simulink model "BFE_TestHarness"  (Simulink 8.6)
settings: Solver=FixedStepDiscrete  StartTime=0.0  StopTime=3  FixedStep=Ts  RelTol=1e-3
PreLoadFcn:
  | addpath('MBD_Tests')
  | 
  | load('Workspace\EnvVar.mat')
  | run('MBD_Tests\MBD_tests_init.m')
  | if exist('tl_preloadfcn','file'), tl_preloadfcn(gcs,402); end
PostLoadFcn:
  | if exist('tl_postloadfcn','file'), tl_postloadfcn(gcs,402); end
InitFcn:
  | if exist('tlds_init','file'), tlds_init(gcs); end
StartFcn:
  | if exist('tlds_start','file'), tlds_start(gcs); end
StopFcn:
  | if exist('tlds_stop','file'), tlds_stop(gcs); end
undefined symbols (not defined in the file): ddv, Ts, u2, u3, u4
libraries: tllib x11, simulink x8, LIB_TF_G_111 x2, LIB_TF_G_12_StepControl x2, LIB_TF_G_112 x1, LIB_TF_G_113 x1
(part 9 of 17)

== system BFE_TestHarness/BFE_AC_BeltFunctionExecution/Subsystem/BFE_AC_BeltFunctionExecution/BFE_AC_BeltFunctionExecution/BFE_runExecuteStandardSteps/ExecuteStandardSteps/SubsystemConvertOrderToMotorPower/Init_Error_Calculation ==
  bIsPRevStepHP : Inport  RequirementInfo={} %GIDa_3aeca3b8_c2ea_4c02_8ac4_92ccbe5190c0
  s8OldPWM : Inport  RequirementInfo={} %GIDa_90f46303_ced5_474c_93d6_f92ab99d1bda  Port=2
  s32OldErrorInteger : Inport  RequirementInfo={} %GIDa_3b3164d8_b308_429e_9a70_7366f48c17f1  Port=3
  Constant : Constant  Value=64  mask(TL_Constant){data={'date',735951.66853295139}}
      settings: CopyFcn=if exist('tl_reset_reviewflag','file')==2,tl_reset_reviewflag(gcbh);end  DeleteFcn=if exist('delete_tlblock','file')==2,delete_tlblock(gcbh);end  NameChangeFcn=if exist('rename_tlblock','file')==2,rename_tlblock(gcbh);end  OpenFcn=if exist('tl_open_blockdlg','file')==2,tl_open_blockdlg(gcbh);else,open_system(gcbh,'parameter');end
      mask Help: eval(['if exist(''tl_online_help'',''file'') == 2, tl_online_help(''Topic'',''TL_Constant''),else, web([''jar:file:///'',matlabroot,''/help/toolbox/simulink/help.jar!/slref/' lower(get_param(gcbh,'Blocktype')) '.html''], ''-helpbrowser''),end'])
      mask Display: plot([-0.05, 1.05, NaN, -0.05, 1.05],[.01, .01, NaN, .99, .99])
  KU16_INIT_INT_ERR_AFTER_HP_STEP : Constant  RequirementInfo={} %GIDa_0c6897e5_41ba_4ffa_a647_dc1e963ab64a  Value=ddv('BFE_Config_Data/KU16_INIT_INT_ERR_AFTER_HP_STEP')  OutDataTypeStr=uint16  mask(TL_Constant){data={'output',{'variable','BFE_Config_Data/KU16_INIT_INT_ERR_AFTER_HP_STEP'},'date',735951.66853256943}}
      settings: CopyFcn=if exist('tl_reset_reviewflag','file')==2,tl_reset_reviewflag(gcbh);end  DeleteFcn=if exist('delete_tlblock','file')==2,delete_tlblock(gcbh);end  NameChangeFcn=if exist('rename_tlblock','file')==2,rename_tlblock(gcbh);end  OpenFcn=if exist('tl_open_blockdlg','file')==2,tl_open_blockdlg(gcbh);else,open_system(gcbh,'parameter');end
      mask Help: eval(['if exist(''tl_online_help'',''file'') == 2, tl_online_help(''Topic'',''TL_Constant''),else, web([''jar:file:///'',matlabroot,''/help/toolbox/simulink/help.jar!/slref/' lower(get_param(gcbh,'Blocktype')) '.html''], ''-helpbrowser''),end'])
      mask Display: plot([-0.05, 1.05, NaN, -0.05, 1.05],[.01, .01, NaN, .99, .99])
  Logical Operator : Logic  RequirementInfo={} %GIDa_e9ae38f0_28a3_485d_bbad_fe83290044bf  Operator=NOT  Inputs=1  AllPortsSameDT=off  OutDataTypeStr=boolean  mask(TL_LogicalOperator){data={'date',735951.66853221064}}
      settings: DeleteFcn=if exist('delete_tlblock','file')==2,delete_tlblock(gcbh);end  NameChangeFcn=if exist('rename_tlblock','file')==2,rename_tlblock(gcbh);end  OpenFcn=if exist('tl_open_blockdlg','file')==2,tl_open_blockdlg(gcbh);else,open_system(gcbh,'parameter');end
      mask Help: eval(['if exist(''tl_online_help'',''file'') == 2, tl_online_help(''Topic'',''TL_LogicalOperator''),else, web([''jar:file:///'',matlabroot,''/help/toolbox/simulink/help.jar!/slref/' lower(get_param(gcbh,'Blocktype')) '.html''], ''-helpbrowser''),end'])
      mask Display: plot([-0.05, 1.05, NaN, -0.05, 1.05],[.01, .01, NaN, .99, .99])
  Product : Product  RequirementInfo={} %GIDa_8a9d49ec_e92b_4899_920d_3eb12938c5eb  Inputs=**  RndMeth=Zero  mask(TL_Product){data={'output',{'type','Int32'},'date',735951.66853192134}}
      settings: CopyFcn=if exist('tl_reset_reviewflag','file')==2,tl_reset_reviewflag(gcbh);end  DeleteFcn=if exist('delete_tlblock','file')==2,delete_tlblock(gcbh);end  NameChangeFcn=if exist('rename_tlblock','file')==2,rename_tlblock(gcbh);end  OpenFcn=if exist('tl_open_blockdlg','file')==2,tl_open_blockdlg(gcbh);else,open_system(gcbh,'parameter');end
      mask Help: eval(['if exist(''tl_online_help'',''file'') == 2, tl_online_help(''Topic'',''TL_Product''),else, web([''jar:file:///'',matlabroot,''/help/toolbox/simulink/help.jar!/slref/' lower(get_param(gcbh,'Blocktype')) '.html''], ''-helpbrowser''),end'])
      mask Display: plot([-0.05, 1.05, NaN, -0.05, 1.05],[.01, .01, NaN, .99, .99])
  Product1 : Product  Inputs=*/  RndMeth=Zero  mask(TL_Product){data={'date',735951.66853155091}}
      settings: CopyFcn=if exist('tl_reset_reviewflag','file')==2,tl_reset_reviewflag(gcbh);end  DeleteFcn=if exist('delete_tlblock','file')==2,delete_tlblock(gcbh);end  NameChangeFcn=if exist('rename_tlblock','file')==2,rename_tlblock(gcbh);end  OpenFcn=if exist('tl_open_blockdlg','file')==2,tl_open_blockdlg(gcbh);else,open_system(gcbh,'parameter');end
      mask Help: eval(['if exist(''tl_online_help'',''file'') == 2, tl_online_help(''Topic'',''TL_Product''),else, web([''jar:file:///'',matlabroot,''/help/toolbox/simulink/help.jar!/slref/' lower(get_param(gcbh,'Blocktype')) '.html''], ''-helpbrowser''),end'])
      mask Display: plot([-0.05, 1.05, NaN, -0.05, 1.05],[.01, .01, NaN, .99, .99])
  Switch2 : Switch  RequirementInfo={} %GIDa_7eaf5a01_1953_49b8_89c4_2db1d6eb7e42  Criteria=u2 ~= 0  mask(TL_Switch){data={'output',{'type','Int32'},'date',735951.66853114578}}
      settings: CopyFcn=if exist('tl_reset_reviewflag','file')==2,tl_reset_reviewflag(gcbh);end  DeleteFcn=if exist('delete_tlblock','file')==2,delete_tlblock(gcbh);end  NameChangeFcn=if exist('rename_tlblock','file')==2,rename_tlblock(gcbh);end  OpenFcn=if exist('tl_open_blockdlg','file')==2,tl_open_blockdlg(gcbh);else,open_system(gcbh,'parameter');end
      mask Help: eval(['if exist(''tl_online_help'',''file'') == 2, tl_online_help(''Topic'',''TL_Switch''),else, web([''jar:file:///'',matlabroot,''/help/toolbox/simulink/help.jar!/slref/' lower(get_param(gcbh,'Blocktype')) '.html''], ''-helpbrowser''),end'])
      mask Display: plot([-0.05, 1.05, NaN, -0.05, 1.05],[.01, .01, NaN, .99, .99])
  s32OldErrorIntegerOut : Outport  RequirementInfo={} %GIDa_0e251ad7_27d7_4147_9d0f_3aab0ebc726c
  wires:
  s32OldErrorInteger/1 -> Switch2/1
  bIsPRevStepHP/1 -> Logical Operator/1
  Logical Operator/1 -> Switch2/2
  Switch2/1 -> s32OldErrorIntegerOut/1
  Product/1 -> Switch2/3
  KU16_INIT_INT_ERR_AFTER_HP_STEP/1 -> Product/2
  Product1/1 -> Product/1
  s8OldPWM/1 -> Product1/1
  Constant/1 -> Product1/2

== system BFE_TestHarness/BFE_AC_BeltFunctionExecution/Subsystem/BFE_AC_BeltFunctionExecution/BFE_AC_BeltFunctionExecution/BFE_runExecuteStandardSteps/ExecuteStandardSteps/SubsystemConvertOrderToMotorPower/ManageIntegerErrorReset ==
  u8OrderType : Inport  RequirementInfo={} %GIDa_8549e3bb_6e62_49c5_b285_24fb3bfbc57d
  s32IntegerErrorBeforeFiltering : Inport  RequirementInfo={} %GIDa_94248635_d0d9_4096_9756_d2821aac4d1d  Port=2
  Constant : Constant  RequirementInfo={} %GIDa_400b47d7_22f6_4b23_999f_d1b51fb3a630  Value=ddv('BFE/Step_Def/KU8_NO_STEP_TYPE')  OutDataTypeStr=uint8  mask(TL_Constant){data={'output',{'variable','BFE/Step_Def/KU8_NO_STEP_TYPE'},'date',735951.66853064811}}
      settings: AttributesFormatString=KUC_ORDER_NO_STEP  CopyFcn=if exist('tl_reset_reviewflag','file')==2,tl_reset_reviewflag(gcbh);end  DeleteFcn=if exist('delete_tlblock','file')==2,delete_tlblock(gcbh);end  NameChangeFcn=if exist('rename_tlblock','file')==2,rename_tlblock(gcbh);end  OpenFcn=if exist('tl_open_blockdlg','file')==2,tl_open_blockdlg(gcbh);else,open_system(gcbh,'parameter');end
      mask Help: eval(['if exist(''tl_online_help'',''file'') == 2, tl_online_help(''Topic'',''TL_Constant''),else, web([''jar:file:///'',matlabroot,''/help/toolbox/simulink/help.jar!/slref/' lower(get_param(gcbh,'Blocktype')) '.html''], ''-helpbrowser''),end'])
      mask Display: plot([-0.05, 1.05, NaN, -0.05, 1.05],[.01, .01, NaN, .99, .99])
  Constant1 : Constant  RequirementInfo={} %GIDa_60b49a3c_45d1_477a_9f0e_42be2507b875  Value=ddv('Common/KU16_ZERO')  OutDataTypeStr=uint16  mask(TL_Constant){data={'output',{'variable','Common/KU16_ZERO'},'date',735951.66853027779}}
      settings: AttributesFormatString=0  CopyFcn=if exist('tl_reset_reviewflag','file')==2,tl_reset_reviewflag(gcbh);end  DeleteFcn=if exist('delete_tlblock','file')==2,delete_tlblock(gcbh);end  NameChangeFcn=if exist('rename_tlblock','file')==2,rename_tlblock(gcbh);end  OpenFcn=if exist('tl_open_blockdlg','file')==2,tl_open_blockdlg(gcbh);else,open_system(gcbh,'parameter');end
      mask Help: eval(['if exist(''tl_online_help'',''file'') == 2, tl_online_help(''Topic'',''TL_Constant''),else, web([''jar:file:///'',matlabroot,''/help/toolbox/simulink/help.jar!/slref/' lower(get_param(gcbh,'Blocktype')) '.html''], ''-helpbrowser''),end'])
      mask Display: plot([-0.05, 1.05, NaN, -0.05, 1.05],[.01, .01, NaN, .99, .99])
  Constant2 : Constant  RequirementInfo={} %GIDa_d35160b3_7e05_486a_a35e_53ff5ad5257b  Value=ddv('Sampling_Freq/KUS_MOTOR_PERIOD')  OutDataTypeStr=uint16  mask(TL_Constant){data={'output',{'variable','Sampling_Freq/KUS_MOTOR_PERIOD'},'date',735951.66852989583}}
      settings: AttributesFormatString=KUS_MOTOR_PERIOD  CopyFcn=if exist('tl_reset_reviewflag','file')==2,tl_reset_reviewflag(gcbh);end  DeleteFcn=if exist('delete_tlblock','file')==2,delete_tlblock(gcbh);end  NameChangeFcn=if exist('rename_tlblock','file')==2,rename_tlblock(gcbh);end  OpenFcn=if exist('tl_open_blockdlg','file')==2,tl_open_blockdlg(gcbh);else,open_system(gcbh,'parameter');end
      mask Help: eval(['if exist(''tl_online_help'',''file'') == 2, tl_online_help(''Topic'',''TL_Constant''),else, web([''jar:file:///'',matlabroot,''/help/toolbox/simulink/help.jar!/slref/' lower(get_param(gcbh,'Blocktype')) '.html''], ''-helpbrowser''),end'])
      mask Display: plot([-0.05, 1.05, NaN, -0.05, 1.05],[.01, .01, NaN, .99, .99])
  Constant3 : Constant  RequirementInfo={} %GIDa_93e02d8c_4049_4a05_a6b4_77b5e0e5f5bc  Value=ddv('BFE_Config_Data/KUS_LATENCY_TIME')  OutDataTypeStr=uint16  mask(TL_Constant){data={'output',{'variable','BFE_Config_Data/KUS_LATENCY_TIME'},'date',735951.66852952552}}
      settings: AttributesFormatString=KUS_LATENCY_TIME  CopyFcn=if exist('tl_reset_reviewflag','file')==2,tl_reset_reviewflag(gcbh);end  DeleteFcn=if exist('delete_tlblock','file')==2,delete_tlblock(gcbh);end  NameChangeFcn=if exist('rename_tlblock','file')==2,rename_tlblock(gcbh);end  OpenFcn=if exist('tl_open_blockdlg','file')==2,tl_open_blockdlg(gcbh);else,open_system(gcbh,'parameter');end
      mask Help: eval(['if exist(''tl_online_help'',''file'') == 2, tl_online_help(''Topic'',''TL_Constant''),else, web([''jar:file:///'',matlabroot,''/help/toolbox/simulink/help.jar!/slref/' lower(get_param(gcbh,'Blocktype')) '.html''], ''-helpbrowser''),end'])
      mask Display: plot([-0.05, 1.05, NaN, -0.05, 1.05],[.01, .01, NaN, .99, .99])
  Constant4 : Constant  RequirementInfo={} %GIDa_677fe65a_1a86_4eeb_a304_f896904fa8d3  Value=ddv('Common/KS32_ZERO')  OutDataTypeStr=int32  mask(TL_Constant){data={'output',{'variable','Common/KS32_ZERO'},'date',735951.66852913192}}
      settings: AttributesFormatString=0  CopyFcn=if exist('tl_reset_reviewflag','file')==2,tl_reset_reviewflag(gcbh);end  DeleteFcn=if exist('delete_tlblock','file')==2,delete_tlblock(gcbh);end  NameChangeFcn=if exist('rename_tlblock','file')==2,rename_tlblock(gcbh);end  OpenFcn=if exist('tl_open_blockdlg','file')==2,tl_open_blockdlg(gcbh);else,open_system(gcbh,'parameter');end
      mask Help: eval(['if exist(''tl_online_help'',''file'') == 2, tl_online_help(''Topic'',''TL_Constant''),else, web([''jar:file:///'',matlabroot,''/help/toolbox/simulink/help.jar!/slref/' lower(get_param(gcbh,'Blocktype')) '.html''], ''-helpbrowser''),end'])
      mask Display: plot([-0.05, 1.05, NaN, -0.05, 1.05],[.01, .01, NaN, .99, .99])
  Relational Operator : RelationalOperator  RequirementInfo={} %GIDa_8dc24057_5624_4d83_81c1_9cda726f5202  Operator===  OutDataTypeStr=boolean  mask(TL_RelationalOperator){data={'date',735951.6685287616}}
      settings: DeleteFcn=if exist('delete_tlblock','file')==2,delete_tlblock(gcbh);end  NameChangeFcn=if exist('rename_tlblock','file')==2,rename_tlblock(gcbh);end  OpenFcn=if exist('tl_open_blockdlg','file')==2,tl_open_blockdlg(gcbh);else,open_system(gcbh,'parameter');end
      mask Help: eval(['if exist(''tl_online_help'',''file'') == 2, tl_online_help(''Topic'',''TL_RelationalOperator''),else, web([''jar:file:///'',matlabroot,''/help/toolbox/simulink/help.jar!/slref/' lower(get_param(gcbh,'Blocktype')) '.html''], ''-helpbrowser''),end'])
      mask Display: plot([-0.05, 1.05, NaN, -0.05, 1.05],[.01, .01, NaN, .99, .99])
  Relational Operator1 : RelationalOperator  RequirementInfo={} %GIDa_358a1e32_d0c5_4061_86ff_eee2b1d5aee8  Operator===  OutDataTypeStr=boolean  mask(TL_RelationalOperator){data={'date',735951.668528507}}
      settings: DeleteFcn=if exist('delete_tlblock','file')==2,delete_tlblock(gcbh);end  NameChangeFcn=if exist('rename_tlblock','file')==2,rename_tlblock(gcbh);end  OpenFcn=if exist('tl_open_blockdlg','file')==2,tl_open_blockdlg(gcbh);else,open_system(gcbh,'parameter');end
      mask Help: eval(['if exist(''tl_online_help'',''file'') == 2, tl_online_help(''Topic'',''TL_RelationalOperator''),else, web([''jar:file:///'',matlabroot,''/help/toolbox/simulink/help.jar!/slref/' lower(get_param(gcbh,'Blocktype')) '.html''], ''-helpbrowser''),end'])
      mask Display: plot([-0.05, 1.05, NaN, -0.05, 1.05],[.01, .01, NaN, .99, .99])
  Saturation : Saturate  RequirementInfo={} %GIDa_0b354fed_29ce_4153_9483_4349c0983084  UpperLimit=ddv('BFE_Config_Data/KUS_LATENCY_TIME')  LowerLimit=ddv('Common/KU16_ZERO')  mask(TL_Saturate){data={'output',{'type','UInt16'},'lowerlimit',{'variable','Common/KU16_ZERO'},'upperlimit',{'variable','BFE_Config_Data/KUS_LATENCY_TIME'},'date',735951.66852819442}}
      settings: CopyFcn=if exist('tl_reset_reviewflag','file')==2,tl_reset_reviewflag(gcbh);end  DeleteFcn=if exist('delete_tlblock','file')==2,delete_tlblock(gcbh);end  NameChangeFcn=if exist('rename_tlblock','file')==2,rename_tlblock(gcbh);end  OpenFcn=if exist('tl_open_blockdlg','file')==2,tl_open_blockdlg(gcbh);else,open_system(gcbh,'parameter');end
      settings: AttributesFormatString=|
      | Lower limit = %<LowerLimit>
      | Upper limit = %<UpperLimit>
      mask Help: eval(['if exist(''tl_online_help'',''file'') == 2, tl_online_help(''Topic'',''TL_Saturate''),else, web([''jar:file:///'',matlabroot,''/help/toolbox/simulink/help.jar!/slref/' lower(get_param(gcbh,'Blocktype')) '.html''], ''-helpbrowser''),end'])
      mask Display: plot([-0.05, 1.05, NaN, -0.05, 1.05],[.01, .01, NaN, .99, .99])
  Sum : Sum  RequirementInfo={} %GIDa_3d53df66_2771_419d_a11b_8bf48d1e7499  mask(TL_Sum){data={'output',{'type','UInt16'},'date',735951.66852752317}}
      settings: CopyFcn=if exist('tl_reset_reviewflag','file')==2,tl_reset_reviewflag(gcbh);end  DeleteFcn=if exist('delete_tlblock','file')==2,delete_tlblock(gcbh);end  NameChangeFcn=if exist('rename_tlblock','file')==2,rename_tlblock(gcbh);end  OpenFcn=if exist('tl_open_blockdlg','file')==2,tl_open_blockdlg(gcbh);else,open_system(gcbh,'parameter');end
      mask Help: eval(['if exist(''tl_online_help'',''file'') == 2, tl_online_help(''Topic'',''TL_Sum''),else, web([''jar:file:///'',matlabroot,''/help/toolbox/simulink/help.jar!/slref/' lower(get_param(gcbh,'Blocktype')) '.html''], ''-helpbrowser''),end'])
      mask Display: plot([-0.05, 1.05, NaN, -0.05, 1.05],[.01, .01, NaN, .99, .99])
  Switch : Switch  RequirementInfo={} %GIDa_fc0b4065_c48a_495e_8057_422aaf68c743  Criteria=u2 ~= 0  mask(TL_Switch){data={'output',{'type','UInt16'},'date',735951.66852712957}}
      settings: CopyFcn=if exist('tl_reset_reviewflag','file')==2,tl_reset_reviewflag(gcbh);end  DeleteFcn=if exist('delete_tlblock','file')==2,delete_tlblock(gcbh);end  NameChangeFcn=if exist('rename_tlblock','file')==2,rename_tlblock(gcbh);end  OpenFcn=if exist('tl_open_blockdlg','file')==2,tl_open_blockdlg(gcbh);else,open_system(gcbh,'parameter');end
      mask Help: eval(['if exist(''tl_online_help'',''file'') == 2, tl_online_help(''Topic'',''TL_Switch''),else, web([''jar:file:///'',matlabroot,''/help/toolbox/simulink/help.jar!/slref/' lower(get_param(gcbh,'Blocktype')) '.html''], ''-helpbrowser''),end'])
      mask Display: plot([-0.05, 1.05, NaN, -0.05, 1.05],[.01, .01, NaN, .99, .99])
  Switch1 : Switch  RequirementInfo={} %GIDa_8f433719_feec_41c9_b899_87ec8cd62b2c  Criteria=u2 ~= 0  mask(TL_Switch){data={'output',{'type','Int32'},'date',735951.6685265972}}
      settings: CopyFcn=if exist('tl_reset_reviewflag','file')==2,tl_reset_reviewflag(gcbh);end  DeleteFcn=if exist('delete_tlblock','file')==2,delete_tlblock(gcbh);end  NameChangeFcn=if exist('rename_tlblock','file')==2,rename_tlblock(gcbh);end  OpenFcn=if exist('tl_open_blockdlg','file')==2,tl_open_blockdlg(gcbh);else,open_system(gcbh,'parameter');end
      mask Help: eval(['if exist(''tl_online_help'',''file'') == 2, tl_online_help(''Topic'',''TL_Switch''),else, web([''jar:file:///'',matlabroot,''/help/toolbox/simulink/help.jar!/slref/' lower(get_param(gcbh,'Blocktype')) '.html''], ''-helpbrowser''),end'])
      mask Display: plot([-0.05, 1.05, NaN, -0.05, 1.05],[.01, .01, NaN, .99, .99])
  Unit Delay : UnitDelay  RequirementInfo={} %GIDa_8c292399_951b_41af_8b19_51277957374b  SampleTime=-1  mask(TL_UnitDelay){data={'output',{'type','UInt16'},'state',{'name','X_u16CntErrorReset','type','UInt16'},'date',735951.66852607636}}
      settings: CopyFcn=if exist('tl_reset_reviewflag','file')==2,tl_reset_reviewflag(gcbh);end  DeleteFcn=if exist('delete_tlblock','file')==2,delete_tlblock(gcbh);end  NameChangeFcn=if exist('rename_tlblock','file')==2,rename_tlblock(gcbh);end  OpenFcn=if exist('tl_open_blockdlg','file')==2,tl_open_blockdlg(gcbh);else,open_system(gcbh,'parameter');end
      mask Help: eval(['if exist(''tl_online_help'',''file'') == 2, tl_online_help(''Topic'',''TL_UnitDelay''),else, web([''jar:file:///'',matlabroot,''/help/toolbox/simulink/help.jar!/slref/' lower(get_param(gcbh,'Blocktype')) '.html''], ''-helpbrowser''),end'])
      mask Display: plot([-0.05, 1.05, NaN, -0.05, 1.05],[.01, .01, NaN, .99, .99])
  s32OldErrorFiltered : Outport  RequirementInfo={} %GIDa_4f4b4710_9940_4364_9238_933101741456
  b8IsNewCycle : Outport  RequirementInfo={} %GIDa_f359d049_9be5_425a_8c81_91d895b874f4  Port=2
  wires:
  u8OrderType/1 -> Relational Operator/1
  Constant/1 -> Relational Operator/2
  Relational Operator/1 -> Switch/2
  Constant1/1 -> Switch/3
  Unit Delay/1 -> Switch/1
  Constant2/1 -> Sum/2
  Switch/1 -> Sum/1
  Sum/1 -> Saturation/1
  Saturation/1 -> Unit Delay/1, Relational Operator1/1
  Constant3/1 -> Relational Operator1/2
  Relational Operator1/1 -> b8IsNewCycle/1, Switch1/2
  s32IntegerErrorBeforeFiltering/1 -> Switch1/3
  Constant4/1 -> Switch1/1
  Switch1/1 -> s32OldErrorFiltered/1

== system BFE_TestHarness/BFE_AC_BeltFunctionExecution/Subsystem/BFE_AC_BeltFunctionExecution/BFE_AC_BeltFunctionExecution/BFE_runExecuteStandardSteps/ExecuteStandardSteps/SubsystemConvertOrderToMotorPower/MotorVoltage_Regulation ==
  lOrderToApply : Inport  RequirementInfo={} %GIDa_276e94c1_4a1d_4441_aa6e_71c39ac6771d
  usBatteryVoltage : Inport  RequirementInfo={} %GIDa_bdb98f1d_8da6_4ac7_8ba3_6dd808cf08bb  Port=2
  Action Port : ActionPort  RequirementInfo={} %GIDa_490740ec_3218_4b5f_9934_5823e2c144e8  ActionType=case
  Battery voltage rescaling : Subsystem  TreatAsAtomicUnit=on
  Consign < Battery voltage => Compute PWM : Subsystem  TreatAsAtomicUnit=on
  Consign > Battery voltage => Saturate to MAX PWM : Subsystem  TreatAsAtomicUnit=on
  If : If  IfExpression=u1
  Implausible order : RelationalOperator  Operator=>  OutDataTypeStr=boolean  mask(TL_RelationalOperator){data={'date',737167.45056728006}}
      settings: DeleteFcn=if exist('delete_tlblock','file')==2,delete_tlblock(gcbh);end  NameChangeFcn=if exist('rename_tlblock','file')==2,rename_tlblock(gcbh);end  OpenFcn=if exist('tl_open_blockdlg','file')==2,tl_open_blockdlg(gcbh);else,open_system(gcbh,'parameter');end
      mask Help: eval(['if exist(''tl_online_help'',''file'') == 2, tl_online_help(''Topic'',''TL_RelationalOperator''),else, web([''jar:file:///'',matlabroot,''/help/toolbox/simulink/help.jar!/slref/' lower(get_param(gcbh,'Blocktype')) '.html''], ''-helpbrowser''),end'])
      mask Display: plot([-0.1, 1.05, NaN, -0.1, 1.05],[.01, .01, NaN, .99, .99]);
  Merge : Merge  mask(TL_Merge){data={'date',737167.47328359948}}
      settings: CopyFcn=if exist('tl_reset_reviewflag') == 2, tl_reset_reviewflag(gcbh); end  DeleteFcn=if exist('delete_tlblock','file')==2,delete_tlblock(gcbh);end  NameChangeFcn=if exist('rename_tlblock','file')==2,rename_tlblock(gcbh);end  OpenFcn=if exist('tl_open_blockdlg','file')==2,tl_open_blockdlg(gcbh);else,open_system(gcbh,'parameter');end
      mask Help: eval(['if exist(''tl_online_help'',''file'') == 2, tl_online_help(''Topic'',''TL_Merge''),else, web([''jar:file:///'',matlabroot,''/help/toolbox/simulink/help.jar!/slref/' lower(get_param(gcbh,'Blocktype')) '.html''], ''-helpbrowser''),end'])
      mask Display: plot([-0.1, 1.05, NaN, -0.1, 1.05],[.01, .01, NaN, .99, .99]);
  RescalerMotorOrder : DataTypeConversion  RequirementInfo={} %GIDa_7ffb3157_f329_4896_ac59_557cf7694e9e  OutDataTypeStr=int16  RndMeth=Zero  mask(TL_Rescaler){data={'output',{'checkmin',1,'checkmax',1},'date',735951.66852125002}}
      settings: DeleteFcn=if exist('delete_tlblock','file')==2,delete_tlblock(gcbh);end  NameChangeFcn=if exist('rename_tlblock','file')==2,rename_tlblock(gcbh);end  OpenFcn=if exist('tl_open_blockdlg','file')==2,tl_open_blockdlg(gcbh);else,open_system(gcbh,'parameter');end
      mask Help: eval(['if exist(''tl_online_help'',''file'') == 2, tl_online_help(''Topic'',''TL_Rescaler''),else, web([''jar:file:///'',matlabroot,''/help/toolbox/simulink/help.jar!/slref/' lower(get_param(gcbh,'Blocktype')) '.html''], ''-helpbrowser''),end'])
      mask Display: plot([-0.05, 1.05, NaN, -0.05, 1.05],[.01, .01, NaN, .99, .99])
  sUnsaturatedMotorPowerOrder : Outport  RequirementInfo={} %GIDa_8479673a_6f27_43fd_8c97_1bdf8f1b517f
  wires:
  RescalerMotorOrder/1 -> sUnsaturatedMotorPowerOrder/1
  lOrderToApply/1 -> Consign > Battery voltage => Saturate to MAX PWM/1(lOrderToApply), Consign < Battery voltage => Compute PWM/1(lOrderToApply), Implausible order/1
  Merge/1 -> RescalerMotorOrder/1
  usBatteryVoltage/1 -> Consign < Battery voltage => Compute PWM/2(usBatteryVoltage), Battery voltage rescaling/1(usBatteryVoltage)
  Battery voltage rescaling/1(usBatteryVoltageScaled) -> Implausible order/2
  Implausible order/1 -> If/1
  If/2 -> Consign < Battery voltage => Compute PWM/Action
  If/1 -> Consign > Battery voltage => Saturate to MAX PWM/Action
  Consign > Battery voltage => Saturate to MAX PWM/1(sUnsaturatedMotorPowerOrder) -> Merge/1
  Consign < Battery voltage => Compute PWM/1(sUnsaturatedMotorPowerOrder) -> Merge/2

== system BFE_TestHarness/BFE_AC_BeltFunctionExecution/Subsystem/BFE_AC_BeltFunctionExecution/BFE_AC_BeltFunctionExecution/BFE_runExecuteStandardSteps/ExecuteStandardSteps/SubsystemConvertOrderToMotorPower/No_Regulation ==
  Action Port : ActionPort  RequirementInfo={} %GIDa_9c14f1c9_1d70_4ac6_acdc_0eeba1f4106a  ActionType=default
  Constant : Constant  RequirementInfo={} %GIDa_3fa52539_92f4_4b6b_8938_fabe1668a03f  Value=ddv('Common/KS16_ZERO')  OutDataTypeStr=int16  mask(TL_Constant){data={'output',{'variable','Common/KS16_ZERO'},'date',735951.66851976851}}
      settings: CopyFcn=if exist('tl_reset_reviewflag','file')==2,tl_reset_reviewflag(gcbh);end  DeleteFcn=if exist('delete_tlblock','file')==2,delete_tlblock(gcbh);end  NameChangeFcn=if exist('rename_tlblock','file')==2,rename_tlblock(gcbh);end  OpenFcn=if exist('tl_open_blockdlg','file')==2,tl_open_blockdlg(gcbh);else,open_system(gcbh,'parameter');end
      mask Help: eval(['if exist(''tl_online_help'',''file'') == 2, tl_online_help(''Topic'',''TL_Constant''),else, web([''jar:file:///'',matlabroot,''/help/toolbox/simulink/help.jar!/slref/' lower(get_param(gcbh,'Blocktype')) '.html''], ''-helpbrowser''),end'])
      mask Display: plot([-0.05, 1.05, NaN, -0.05, 1.05],[.01, .01, NaN, .99, .99])
  Rescaler : DataTypeConversion  RequirementInfo={} %GIDa_7c165c89_8161_486a_8381_b07b38254a18  OutDataTypeStr=int16  SaturateOnIntegerOverflow=on  RndMeth=Zero  mask(TL_Rescaler){data={'date',735951.66851938656}}
      settings: DeleteFcn=if exist('delete_tlblock','file')==2,delete_tlblock(gcbh);end  NameChangeFcn=if exist('rename_tlblock','file')==2,rename_tlblock(gcbh);end  OpenFcn=if exist('tl_open_blockdlg','file')==2,tl_open_blockdlg(gcbh);else,open_system(gcbh,'parameter');end
      mask Help: eval(['if exist(''tl_online_help'',''file'') == 2, tl_online_help(''Topic'',''TL_Rescaler''),else, web([''jar:file:///'',matlabroot,''/help/toolbox/simulink/help.jar!/slref/' lower(get_param(gcbh,'Blocktype')) '.html''], ''-helpbrowser''),end'])
      mask Display: plot([-0.05, 1.05, NaN, -0.05, 1.05],[.01, .01, NaN, .99, .99])
  s16Consign : Outport  RequirementInfo={} %GIDa_00325fa2_2d83_40ec_a061_c69647143619  InitialOutput=0
  wires:
  Constant/1 -> Rescaler/1
  Rescaler/1 -> s16Consign/1

== system BFE_TestHarness/BFE_AC_BeltFunctionExecution/Subsystem/BFE_AC_BeltFunctionExecution/BFE_AC_BeltFunctionExecution/BFE_runExecuteStandardSteps/ExecuteStandardSteps/SubsystemConvertOrderToMotorPower/PWM_Regulation ==
  s32OrderToApply : Inport  RequirementInfo={} %GIDa_80e886a0_f1c3_49a4_98c6_efd74da0210c
  Action Port : ActionPort  RequirementInfo={} %GIDa_d2103cf1_dcab_4113_8a19_04aa9c62073a  ActionType=case
  Arrondi 1/2 lsb : Constant  Value=ddv('BFE/ExecuteStdSteps_Rescaling/KU16_PWM_RSC_NUM')  mask(TL_Constant){data={'output',{'variable','BFE/ExecuteStdSteps_Rescaling/KU16_PWM_RSC_NUM'},'date',735951.6685190741}}
      settings: CopyFcn=if exist('tl_reset_reviewflag','file')==2,tl_reset_reviewflag(gcbh);end  DeleteFcn=if exist('delete_tlblock','file')==2,delete_tlblock(gcbh);end  NameChangeFcn=if exist('rename_tlblock','file')==2,rename_tlblock(gcbh);end  OpenFcn=if exist('tl_open_blockdlg','file')==2,tl_open_blockdlg(gcbh);else,open_system(gcbh,'parameter');end
      mask Help: eval(['if exist(''tl_online_help'',''file'') == 2, tl_online_help(''Topic'',''TL_Constant''),else, web([''jar:file:///'',matlabroot,''/help/toolbox/simulink/help.jar!/slref/' lower(get_param(gcbh,'Blocktype')) '.html''], ''-helpbrowser''),end'])
      mask Display: plot([-0.05, 1.05, NaN, -0.05, 1.05],[.01, .01, NaN, .99, .99])
  Divider to rescale output : Constant  Value=ddv('BFE/ExecuteStdSteps_Rescaling/KU16_PWM_RSC_DEN')  mask(TL_Constant){data={'output',{'variable','BFE/ExecuteStdSteps_Rescaling/KU16_PWM_RSC_DEN'},'date',735951.66851871531}}
      settings: CopyFcn=if exist('tl_reset_reviewflag','file')==2,tl_reset_reviewflag(gcbh);end  DeleteFcn=if exist('delete_tlblock','file')==2,delete_tlblock(gcbh);end  NameChangeFcn=if exist('rename_tlblock','file')==2,rename_tlblock(gcbh);end  OpenFcn=if exist('tl_open_blockdlg','file')==2,tl_open_blockdlg(gcbh);else,open_system(gcbh,'parameter');end
      mask Help: eval(['if exist(''tl_online_help'',''file'') == 2, tl_online_help(''Topic'',''TL_Constant''),else, web([''jar:file:///'',matlabroot,''/help/toolbox/simulink/help.jar!/slref/' lower(get_param(gcbh,'Blocktype')) '.html''], ''-helpbrowser''),end'])
      mask Display: plot([-0.05, 1.05, NaN, -0.05, 1.05],[.01, .01, NaN, .99, .99])
  Product : Product  Inputs=**  RndMeth=Zero  mask(TL_Product){data={'output',{'type','Int32'},'date',735951.66851832171}}
      settings: CopyFcn=if exist('tl_reset_reviewflag','file')==2,tl_reset_reviewflag(gcbh);end  DeleteFcn=if exist('delete_tlblock','file')==2,delete_tlblock(gcbh);end  NameChangeFcn=if exist('rename_tlblock','file')==2,rename_tlblock(gcbh);end  OpenFcn=if exist('tl_open_blockdlg','file')==2,tl_open_blockdlg(gcbh);else,open_system(gcbh,'parameter');end
      mask Help: eval(['if exist(''tl_online_help'',''file'') == 2, tl_online_help(''Topic'',''TL_Product''),else, web([''jar:file:///'',matlabroot,''/help/toolbox/simulink/help.jar!/slref/' lower(get_param(gcbh,'Blocktype')) '.html''], ''-helpbrowser''),end'])
      mask Display: plot([-0.05, 1.05, NaN, -0.05, 1.05],[.01, .01, NaN, .99, .99])
  Product1 : Product  Inputs=*/  RndMeth=Zero  mask(TL_Product){data={'output',{'name','s32PwmConsignBeforeSat','type','Int32'},'date',735951.66851795139}}
      settings: CopyFcn=if exist('tl_reset_reviewflag','file')==2,tl_reset_reviewflag(gcbh);end  DeleteFcn=if exist('delete_tlblock','file')==2,delete_tlblock(gcbh);end  NameChangeFcn=if exist('rename_tlblock','file')==2,rename_tlblock(gcbh);end  OpenFcn=if exist('tl_open_blockdlg','file')==2,tl_open_blockdlg(gcbh);else,open_system(gcbh,'parameter');end
      mask Help: eval(['if exist(''tl_online_help'',''file'') == 2, tl_online_help(''Topic'',''TL_Product''),else, web([''jar:file:///'',matlabroot,''/help/toolbox/simulink/help.jar!/slref/' lower(get_param(gcbh,'Blocktype')) '.html''], ''-helpbrowser''),end'])
      mask Display: plot([-0.05, 1.05, NaN, -0.05, 1.05],[.01, .01, NaN, .99, .99])
  Rescaler : DataTypeConversion  RequirementInfo={} %GIDa_e673e2b5_0cd4_4efe_a1c1_bc5c66dccb61  OutDataTypeStr=int16  RndMeth=Zero  mask(TL_Rescaler){data={'output',{'checkmin',1,'checkmax',1},'date',735951.66851761576}}
      settings: DeleteFcn=if exist('delete_tlblock','file')==2,delete_tlblock(gcbh);end  NameChangeFcn=if exist('rename_tlblock','file')==2,rename_tlblock(gcbh);end  OpenFcn=if exist('tl_open_blockdlg','file')==2,tl_open_blockdlg(gcbh);else,open_system(gcbh,'parameter');end
      mask Help: eval(['if exist(''tl_online_help'',''file'') == 2, tl_online_help(''Topic'',''TL_Rescaler''),else, web([''jar:file:///'',matlabroot,''/help/toolbox/simulink/help.jar!/slref/' lower(get_param(gcbh,'Blocktype')) '.html''], ''-helpbrowser''),end'])
      mask Display: plot([-0.05, 1.05, NaN, -0.05, 1.05],[.01, .01, NaN, .99, .99])
  Sign : Signum  mask(TL_Signum){data={'output',{'name','s16TargetSign_$S'},'date',735951.66851730319}}
      settings: DeleteFcn=if exist('delete_tlblock','file')==2,delete_tlblock(gcbh);end  NameChangeFcn=if exist('rename_tlblock','file')==2,rename_tlblock(gcbh);end  OpenFcn=if exist('tl_open_blockdlg','file')==2,tl_open_blockdlg(gcbh);else,open_system(gcbh,'parameter');end
      mask Help: eval(['if exist(''tl_online_help'',''file'') == 2, tl_online_help(''Topic'',''TL_Signum''),else, web([''jar:file:///'',matlabroot,''/help/toolbox/simulink/help.jar!/slref/' lower(get_param(gcbh,'Blocktype')) '.html''], ''-helpbrowser''),end'])
      mask Display: plot([-0.05, 1.05, NaN, -0.05, 1.05],[.01, .01, NaN, .99, .99])
  Sum : Sum  mask(TL_Sum){data={'output',{'type','Int32'},'date',735951.66851703706}}
      settings: CopyFcn=if exist('tl_reset_reviewflag','file')==2,tl_reset_reviewflag(gcbh);end  DeleteFcn=if exist('delete_tlblock','file')==2,delete_tlblock(gcbh);end  NameChangeFcn=if exist('rename_tlblock','file')==2,rename_tlblock(gcbh);end  OpenFcn=if exist('tl_open_blockdlg','file')==2,tl_open_blockdlg(gcbh);else,open_system(gcbh,'parameter');end
      mask Help: eval(['if exist(''tl_online_help'',''file'') == 2, tl_online_help(''Topic'',''TL_Sum''),else, web([''jar:file:///'',matlabroot,''/help/toolbox/simulink/help.jar!/slref/' lower(get_param(gcbh,'Blocktype')) '.html''], ''-helpbrowser''),end'])
      mask Display: plot([-0.05, 1.05, NaN, -0.05, 1.05],[.01, .01, NaN, .99, .99])
  s16Consign : Outport  RequirementInfo={} %GIDa_f5bdba62_5438_4799_a05e_dd94e80fe2ec  InitialOutput=0
  wires:
  s32OrderToApply/1 -> Sign/1, Sum/2
  Sign/1 -> Product/2
  Product/1 -> Sum/1
  Arrondi 1/2 lsb/1 -> Product/1
  Sum/1 -> Product1/1
  Divider to rescale output/1 -> Product1/2
  Product1/1 -> Rescaler/1
  Rescaler/1 -> s16Consign/1

== system BFE_TestHarness/BFE_AC_BeltFunctionExecution/Subsystem/BFE_AC_BeltFunctionExecution/BFE_AC_BeltFunctionExecution/BFE_runExecuteStandardSteps/ExecuteStandardSteps/SubsystemConvertOrderToMotorPower/RescaleOrderType ==
  u8OrderType : Inport  RequirementInfo={} %GIDa_c5857566_eec0_4dde_a1b4_93ea07e95cd2
  If Action Subsystem : Subsystem  TreatAsAtomicUnit=on
  If Action Subsystem1 : Subsystem  TreatAsAtomicUnit=on
  Merge : Merge  InitialOutput=7  mask(TL_Merge){data={'output',{'name','u8OrderTypeRescaled'},'date',735951.66850811348}}
      settings: CopyFcn=if exist('tl_reset_reviewflag','file')==2,tl_reset_reviewflag(gcbh);end  DeleteFcn=if exist('delete_tlblock','file')==2,delete_tlblock(gcbh);end  NameChangeFcn=if exist('rename_tlblock','file')==2,rename_tlblock(gcbh);end  OpenFcn=if exist('tl_open_blockdlg','file')==2,tl_open_blockdlg(gcbh);else,open_system(gcbh,'parameter');end
      mask Help: eval(['if exist(''tl_online_help'',''file'') == 2, tl_online_help(''Topic'',''TL_Merge''),else, web([''jar:file:///'',matlabroot,''/help/toolbox/simulink/help.jar!/slref/' lower(get_param(gcbh,'Blocktype')) '.html''], ''-helpbrowser''),end'])
      mask Display: plot([-0.05, 1.05, NaN, -0.05, 1.05],[.01, .01, NaN, .99, .99])
  Merge1 : Merge  InitialOutput=0  mask(TL_Merge){data={'output',{'name','bIsSelectedPIDm'},'date',735951.66850771988}}
      settings: CopyFcn=if exist('tl_reset_reviewflag','file')==2,tl_reset_reviewflag(gcbh);end  DeleteFcn=if exist('delete_tlblock','file')==2,delete_tlblock(gcbh);end  NameChangeFcn=if exist('rename_tlblock','file')==2,rename_tlblock(gcbh);end  OpenFcn=if exist('tl_open_blockdlg','file')==2,tl_open_blockdlg(gcbh);else,open_system(gcbh,'parameter');end
      mask Help: eval(['if exist(''tl_online_help'',''file'') == 2, tl_online_help(''Topic'',''TL_Merge''),else, web([''jar:file:///'',matlabroot,''/help/toolbox/simulink/help.jar!/slref/' lower(get_param(gcbh,'Blocktype')) '.html''], ''-helpbrowser''),end'])
      mask Display: plot([-0.05, 1.05, NaN, -0.05, 1.05],[.01, .01, NaN, .99, .99])
  Merge2 : Merge  InitialOutput=0  mask(TL_Merge){data={'output',{'name','bIsSelectedPIDs'},'date',735951.66850732639}}
      settings: CopyFcn=if exist('tl_reset_reviewflag','file')==2,tl_reset_reviewflag(gcbh);end  DeleteFcn=if exist('delete_tlblock','file')==2,delete_tlblock(gcbh);end  NameChangeFcn=if exist('rename_tlblock','file')==2,rename_tlblock(gcbh);end  OpenFcn=if exist('tl_open_blockdlg','file')==2,tl_open_blockdlg(gcbh);else,open_system(gcbh,'parameter');end
      mask Help: eval(['if exist(''tl_online_help'',''file'') == 2, tl_online_help(''Topic'',''TL_Merge''),else, web([''jar:file:///'',matlabroot,''/help/toolbox/simulink/help.jar!/slref/' lower(get_param(gcbh,'Blocktype')) '.html''], ''-helpbrowser''),end'])
      mask Display: plot([-0.05, 1.05, NaN, -0.05, 1.05],[.01, .01, NaN, .99, .99])
  PID Config Preprocessor : Constant  RequirementInfo={} %GIDa_e5ccb42c_0df8_4371_b593_9bc4a20de724  SampleTime=-1  mask(TL_Constant){data={'output',{'variable','BFE_Config_PreProc/BFE_CFG_OPT_PID'},'date',735951.66850695596}}
      settings: CopyFcn=if exist('tl_reset_reviewflag','file')==2,tl_reset_reviewflag(gcbh);end  DeleteFcn=if exist('delete_tlblock','file')==2,delete_tlblock(gcbh);end  NameChangeFcn=if exist('rename_tlblock','file')==2,rename_tlblock(gcbh);end  OpenFcn=if exist('tl_open_blockdlg','file')==2,tl_open_blockdlg(gcbh);else,open_system(gcbh,'parameter');end
      mask Help: eval(['if exist(''tl_online_help'',''file'') == 2, tl_online_help(''Topic'',''TL_Constant''),else, web([''jar:file:///'',matlabroot,''/help/toolbox/simulink/help.jar!/slref/' lower(get_param(gcbh,'Blocktype')) '.html''], ''-helpbrowser''),end'])
      mask Display: plot([-0.05, 1.05, NaN, -0.05, 1.05],[.01, .01, NaN, .99, .99])
  Preprocessor IF : If  RequirementInfo={} %GIDa_c4e4d68b_f4ed_4fdc_b5ff_f174c38962ab  IfExpression=u1  mask(TL_PreProcessorIf){data={'mode',2,'date',735951.6685066435}}
      settings: DeleteFcn=if exist('delete_tlblock','file')==2,delete_tlblock(gcbh);end  NameChangeFcn=if exist('rename_tlblock','file')==2,rename_tlblock(gcbh);end  OpenFcn=if exist('tl_open_blockdlg','file')==2,tl_open_blockdlg(gcbh);else,open_system(gcbh,'parameter');end
      mask Help: eval(['if exist(''tl_online_help'',''file'') == 2, tl_online_help(''Topic'',''TL_PreProcessorIf''),else, web([''jar:file:///'',matlabroot,''/help/toolbox/simulink/help.jar!/slref/' lower(get_param(gcbh,'Blocktype')) '.html''], ''-helpbrowser''),end'])
      mask Display:
      | plot([-0.05, 1.05, NaN, -0.05, 1.05],[.01, .01, NaN, .99, .99])
      | 
      | port_label('input', 1, 'u1')
      | port_label('output',1,'#ifdef u1');
      | port_label('output',2,'#else');
  OrderType_Rescaled : Outport  RequirementInfo={} %GIDa_571aea4a_80c2_4a5a_aedc_995740255ca2
  bIsPID_M : Outport  RequirementInfo={} %GIDa_32a1635e_b6b3_4e10_ade1_227b81beb534  Port=2
  IsPID_S : Outport  RequirementInfo={} %GIDa_9aba60ee_92a3_4f2d_ab51_c6f79f96a8a7  Port=3
  wires:
  PID Config Preprocessor/1 -> Preprocessor IF/1
  Merge/1 -> OrderType_Rescaled/1
  Merge1/1 -> bIsPID_M/1
  Merge2/1 -> IsPID_S/1
  Preprocessor IF/1 -> If Action Subsystem/Action
  Preprocessor IF/2 -> If Action Subsystem1/Action
  u8OrderType/1 -> If Action Subsystem/1(In1), If Action Subsystem1/1(In1)
  If Action Subsystem/1(OrderType_Rescaled) -> Merge/1
  If Action Subsystem/2(bIsPID_M) -> Merge1/1
  If Action Subsystem/3(IsPID_S) -> Merge2/1
  If Action Subsystem1/1(OrderType_Rescaled) -> Merge/2
  If Action Subsystem1/2(bIsPID_M) -> Merge1/2
  If Action Subsystem1/3(IsPID_S) -> Merge2/2

== system BFE_TestHarness/BFE_AC_BeltFunctionExecution/Subsystem/BFE_AC_BeltFunctionExecution/BFE_AC_BeltFunctionExecution/BFE_runExecuteStandardSteps/ExecuteStandardSteps/SubsystemUpdateConsigns/SubsystemDetectConsignsChange ==
  lFirstOrder : Inport  RequirementInfo={} %GIDa_db74001a_2666_4c31_aab5_f76ef3bd28c7
  lIncrement : Inport  RequirementInfo={} %GIDa_477c4fa7_fcac_4b22_9d64_4a2c90d18339  Port=2
  Relational Operator : RelationalOperator  RequirementInfo={} %GIDa_4fa6c098_95de_4c27_8d70_e73712a5e2bb  Operator=~=  OutDataTypeStr=boolean  mask(TL_RelationalOperator){data={'date',735951.66850440972}}
      settings: DeleteFcn=if exist('delete_tlblock','file')==2,delete_tlblock(gcbh);end  NameChangeFcn=if exist('rename_tlblock','file')==2,rename_tlblock(gcbh);end  OpenFcn=if exist('tl_open_blockdlg','file')==2,tl_open_blockdlg(gcbh);else,open_system(gcbh,'parameter');end
      mask Help: eval(['if exist(''tl_online_help'',''file'') == 2, tl_online_help(''Topic'',''TL_RelationalOperator''),else, web([''jar:file:///'',matlabroot,''/help/toolbox/simulink/help.jar!/slref/' lower(get_param(gcbh,'Blocktype')) '.html''], ''-helpbrowser''),end'])
      mask Display: plot([-0.05, 1.05, NaN, -0.05, 1.05],[.01, .01, NaN, .99, .99])
  Relational Operator1 : RelationalOperator  RequirementInfo={} %GIDa_94e3bf36_77c8_4be0_bbfa_11cc96654526  Operator=~=  OutDataTypeStr=boolean  mask(TL_RelationalOperator){data={'output',{'name','bHasFirstOrderChanged'},'date',735951.66850414348}}
      settings: DeleteFcn=if exist('delete_tlblock','file')==2,delete_tlblock(gcbh);end  NameChangeFcn=if exist('rename_tlblock','file')==2,rename_tlblock(gcbh);end  OpenFcn=if exist('tl_open_blockdlg','file')==2,tl_open_blockdlg(gcbh);else,open_system(gcbh,'parameter');end
      mask Help: eval(['if exist(''tl_online_help'',''file'') == 2, tl_online_help(''Topic'',''TL_RelationalOperator''),else, web([''jar:file:///'',matlabroot,''/help/toolbox/simulink/help.jar!/slref/' lower(get_param(gcbh,'Blocktype')) '.html''], ''-helpbrowser''),end'])
      mask Display: plot([-0.05, 1.05, NaN, -0.05, 1.05],[.01, .01, NaN, .99, .99])
  Unit Delay : UnitDelay  RequirementInfo={} %GIDa_93cb41a2_828f_4917_b6f8_88a63358c40e  SampleTime=-1  mask(TL_UnitDelay){data={'output',{'type','Int32'},'state',{'name','s32PrevSlopeValue2ms','type','Int32'},'date',735951.66850384255}}
      settings: CopyFcn=if exist('tl_reset_reviewflag','file')==2,tl_reset_reviewflag(gcbh);end  DeleteFcn=if exist('delete_tlblock','file')==2,delete_tlblock(gcbh);end  NameChangeFcn=if exist('rename_tlblock','file')==2,rename_tlblock(gcbh);end  OpenFcn=if exist('tl_open_blockdlg','file')==2,tl_open_blockdlg(gcbh);else,open_system(gcbh,'parameter');end
      mask Help: eval(['if exist(''tl_online_help'',''file'') == 2, tl_online_help(''Topic'',''TL_UnitDelay''),else, web([''jar:file:///'',matlabroot,''/help/toolbox/simulink/help.jar!/slref/' lower(get_param(gcbh,'Blocktype')) '.html''], ''-helpbrowser''),end'])
      mask Display: plot([-0.05, 1.05, NaN, -0.05, 1.05],[.01, .01, NaN, .99, .99])
  Unit Delay1 : UnitDelay  RequirementInfo={} %GIDa_d0f23ad1_0241_445b_ab17_343554da16e2  SampleTime=-1  mask(TL_UnitDelay){data={'output',{'type','Int32'},'state',{'name','s32PrevFirstValue2ms','type','Int32'},'date',735951.66850331018}}
      settings: CopyFcn=if exist('tl_reset_reviewflag','file')==2,tl_reset_reviewflag(gcbh);end  DeleteFcn=if exist('delete_tlblock','file')==2,delete_tlblock(gcbh);end  NameChangeFcn=if exist('rename_tlblock','file')==2,rename_tlblock(gcbh);end  OpenFcn=if exist('tl_open_blockdlg','file')==2,tl_open_blockdlg(gcbh);else,open_system(gcbh,'parameter');end
      mask Help: eval(['if exist(''tl_online_help'',''file'') == 2, tl_online_help(''Topic'',''TL_UnitDelay''),else, web([''jar:file:///'',matlabroot,''/help/toolbox/simulink/help.jar!/slref/' lower(get_param(gcbh,'Blocktype')) '.html''], ''-helpbrowser''),end'])
      mask Display: plot([-0.05, 1.05, NaN, -0.05, 1.05],[.01, .01, NaN, .99, .99])
  bAreConsignsChanged : Logic  RequirementInfo={} %GIDa_6edf0bbf_29de_40bd_80a3_614c304e4df3  Operator=OR  AllPortsSameDT=off  OutDataTypeStr=boolean  mask(TL_LogicalOperator){data={'output',{'name','$B'},'date',736391.53670037037}}
      settings: DeleteFcn=if exist('delete_tlblock','file')==2,delete_tlblock(gcbh);end  NameChangeFcn=if exist('rename_tlblock','file')==2,rename_tlblock(gcbh);end  OpenFcn=if exist('tl_open_blockdlg','file')==2,tl_open_blockdlg(gcbh);else,open_system(gcbh,'parameter');end
      mask Help: eval(['if exist(''tl_online_help'',''file'') == 2, tl_online_help(''Topic'',''TL_LogicalOperator''),else, web([''jar:file:///'',matlabroot,''/help/toolbox/simulink/help.jar!/slref/' lower(get_param(gcbh,'Blocktype')) '.html''], ''-helpbrowser''),end'])
      mask Display: plot([-0.05, 1.05, NaN, -0.05, 1.05],[.01, .01, NaN, .99, .99])
  bAreConsignsChanged_out : Outport  RequirementInfo={} %GIDa_fb18fe53_8047_449b_b346_4ab8fff4a80e
  wires:
  Relational Operator1/1 -> bAreConsignsChanged/2
  Relational Operator/1 -> bAreConsignsChanged/1
  bAreConsignsChanged/1 -> bAreConsignsChanged_out/1
  Unit Delay1/1 -> Relational Operator1/2
  Unit Delay/1 -> Relational Operator/2
  lIncrement/1 -> Unit Delay/1, Relational Operator/1
  lFirstOrder/1 -> Unit Delay1/1, Relational Operator1/1
